simulink model "ModelC"  (R2014a)
settings: Solver=FixedStepDiscrete  StartTime=0.0  StopTime=10.0  RelTol=1e-3
libraries: simulink x1
settings Model: SimulationMode=external  ExtModeTrigDuration=100  Creator=admin  LastModifiedBy=admin
settings SolverCC: AutoInsertRateTranBlk=on
settings DataIOCC: SaveOutput=off  SaveTime=off
settings OptimizationCC: InlineParams=on  InlineInvariantSignals=on  StateBitsets=on  DataBitsets=on  UseTempVars=on  ZeroExternalMemoryAtStartup=off  ZeroInternalMemoryAtStartup=off  NoFixptDivByZeroProtection=on  EfficientFloat2IntCast=on  OptimizeModelRefInitCode=on  LifeSpan=1
settings DebuggingCC: SolverPrmCheckMsg=none
settings HardwareCC: ProdIntDivRoundTo=Floor  ProdEndianess=LittleEndian  ProdHWDeviceType=Generic->Custom
settings RTWCC: SystemTargetFile=ert.tlc  TLCOptions=-p0  GenCodeOnly=on  TemplateMakefile=ert_default_tmf  Description=Embedded Coder  GenerateReport=on  RTWVerbose=off  ProcessScript=ert_make_rtw_hook  IncludeHyperlinkInReport=on  LaunchReport=on  GenerateTraceInfo=on  GenerateTraceReport=on  GenerateTraceReportSl=on  GenerateTraceReportSf=on  GenerateTraceReportEml=on
settings CodeAppCC: ForceParamTrailComments=on  IgnoreCustomStorageClasses=off  SimulinkDataObjDesc=on  CustomSymbolStrGlobalVar=rt$N$M  CustomSymbolStrType=$N$M  CustomSymbolStrFcn=$N$M$F  CustomSymbolStrMacro=$N$M  InsertBlockDesc=on
settings ERTTargetCC: CodeReplacementLibrary=ISO_C  ParMdlRefBuildCompliant=on  CompOptLevelCompliant=on  ConcurrentExecutionCompliant=on  IncludeMdlTerminateFcn=off  SuppressErrorStatus=on  ERTFirstTimeCompliant=on  SupportAbsoluteTime=off  SupportNonFinite=off  SupportComplex=off  PurelyIntegerCode=on  ModelStepFunctionPrototypeControlCompliant=on  CPPClassGenCompliant=on  RootIOFormat=Structure reference  ERTCustomFileTemplate=example_file_process.tlc

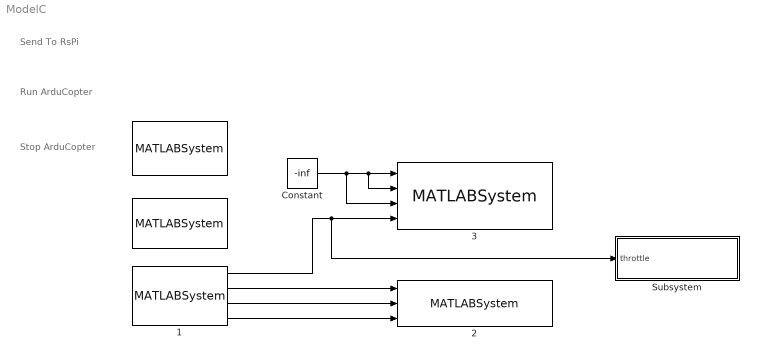
== system ModelC ==
  note: Send To RsPi
  note: Run ArduCopter
  note: Stop ArduCopter
  "  " : MATLABSystem  System=Gyro  SimulateUsing=Interpreted execution
      mask Type: Gyro
      mask Display:
      | disp('Gyro');
      | port_label('output',1,'x');
      | port_label('output',2,'y');
      | port_label('output',3,'z');
  "   " : MATLABSystem  System=Accel  SimulateUsing=Interpreted execution
      mask Type: Accel
      mask Display:
      | disp('Accel');
      | port_label('output',1,'x');
      | port_label('output',2,'y');
      | port_label('output',3,'z');
  "   1" : MATLABSystem  System=RC  SimulateUsing=Interpreted execution
      mask Type: RC
      mask Display:
      | disp('RC');
      | port_label('output',1,'thort');
      | port_label('output',2,'yawR');
      | port_label('output',3,'pitch');
      | port_label('output',4,'roll');
  "   2" : MATLABSystem  System=RateController  SimulateUsing=Interpreted execution
      mask Type: RateController
      mask Display:
      | disp('RateController');
      | port_label('input',1,'yaw');
      | port_label('input',2,'pitch');
      | port_label('input',3,'roll');
  "   3" : MATLABSystem  System=Motors  SimulateUsing=Interpreted execution
      mask Type: Motors
      mask Display:
      | disp('Motors');
      | port_label('input',1,'roll');
      | port_label('input',2,'pitch');
      | port_label('input',3,'yaw');
      | port_label('input',4,'throttle');
  Constant : Constant  Value=-inf
  Subsystem : Subsystem
      mask Display: fprintf('Check throttle range')
  wires:
  "   1"/2 -> "   2"/1
  "   1"/4 -> "   2"/3
  "   1"/3 -> "   2"/2
  Constant/1 -> "   3"/3, "   3"/2, "   3"/1
  "   1"/1 -> Subsystem/1(throttle), "   3"/4

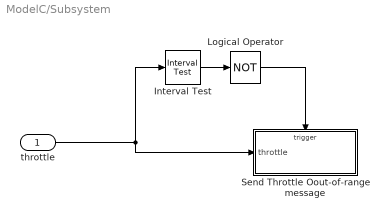
== system ModelC/Subsystem ==
  throttle : Inport
  Interval Test : simulink/Logic and Bit Operations/Interval Test  IntervalClosedRight=on  uplimit=0  IntervalClosedLeft=on  lowlimit=1  OutDataTypeStr=boolean
  Logical Operator : Logic  Operator=NOT  AllPortsSameDT=off  OutDataTypeStr=boolean
  Send Throttle Oout-of-range message : Subsystem  TreatAsAtomicUnit=on
  wires:
  throttle/1 -> Interval Test/1, Send Throttle Oout-of-range message/1(throttle)
  Logical Operator/1 -> Send Throttle Oout-of-range message/Trigger
  Interval Test/1 -> Logical Operator/1

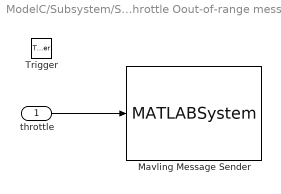
== system ModelC/Subsystem/Send Throttle Oout-of-range message ==
  throttle : Inport
  Trigger : TriggerPort
  Mavling Message Sender : MATLABSystem  System=MavlinkMsg  Message=throttle not between 0 to 1:
      mask Type: MavlinkMsg
      mask Display:
      | disp('MavlinkMsg');
      | port_label('input',1,'u');
  wires:
  throttle/1 -> Mavling Message Sender/1
